simulink model "chap1_8"  (Simulink 3.00)
settings: Solver=ode4  StartTime=0.0  StopTime=2  RelTol=1e-3
settings Model: SaveTime=off  SaveOutput=off  Decimation=100

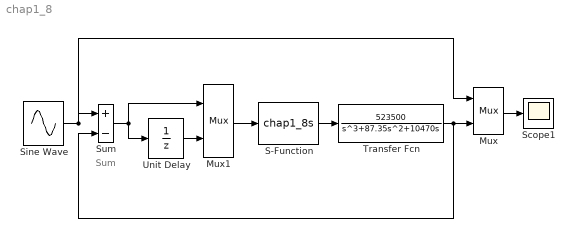
== system chap1_8 ==
  note: Sum
  Mux : Mux  Inputs=2
      settings: DisplayOption=none
  Mux1 : Mux  Inputs=2
      settings: DisplayOption=none
  S-Function : S-Function  FunctionName=chap1_8s  PortCounts=[]  SFunctionModules=''
  Scope1 : Scope
      settings: TimeRange=0.2  YMin=-0.051  YMax=-0.041  SaveToWorkspace=off  SaveName=ScopeData  MaxRows=50000  Decimation=0.001  SampleInput=on  SampleTime=0.001
  Sine Wave : Sin  Amplitude=1  Frequency=1*2*pi  Phase=0  SampleTime=0.001
  Sum : Sum  Inputs=|+-  SaturateOnIntegerOverflow=on
  Transfer Fcn : TransferFcn  Numerator=[523500]  Denominator=[1 87.35 10470 0]
  Unit Delay : UnitDelay  X0=0  SampleTime=0.001
  wires:
  Sine Wave/1 -> Sum/1, Mux/1
  Mux1/1 -> S-Function/1
  Unit Delay/1 -> Mux1/2
  Sum/1 -> Mux1/1, Unit Delay/1
  S-Function/1 -> Transfer Fcn/1
  Mux/1 -> Scope1/1
  Transfer Fcn/1 -> Mux/2, Sum/2
